simulink model "ModelGreenhouse"  (R2018a)
settings: Solver=FixedStepAuto  StartTime=0  StopTime=432000  FixedStep=5  RelTol=1e-1
undefined symbols (not defined in the file or in its folder): magnitude
libraries: simulink x6
(part 1 of 3)
settings Model: SimulationMode=accelerator  Creator=kayfr  LastModifiedBy=kayfr
settings SolverCC: MaxConsecutiveMinStep=100  AlgebraicLoopSolver=LineSearch
settings DebuggingCC: IgnoredZcDiagnostic=none

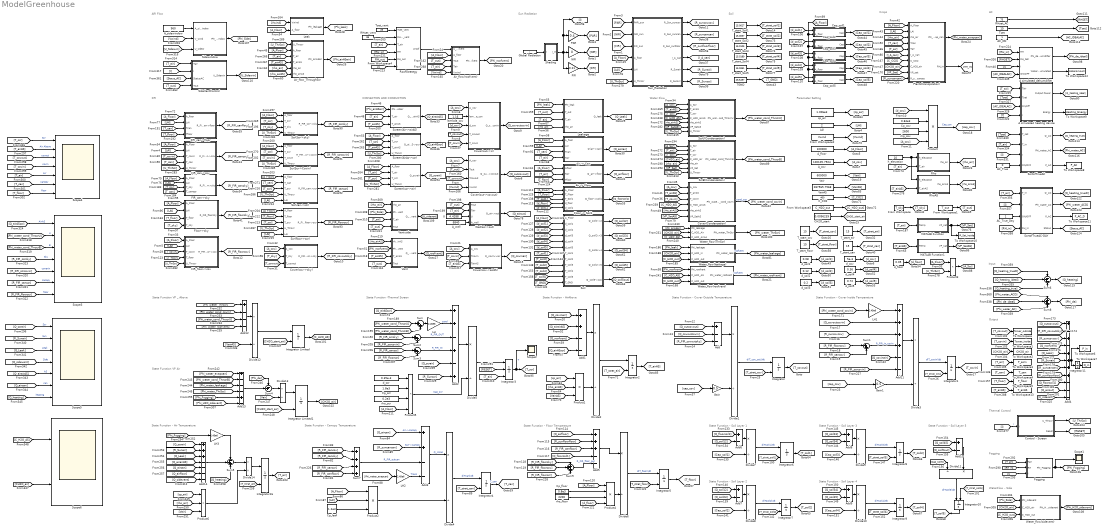
== system ModelGreenhouse ==
  note: Input
  note: AC
  note: WaterFlow - Side
  note: Fogging
  note: Thermal Control
  note: State Function - Air Temperature
  note: State Function VP Air
  note: State Function VP _ Above
  note: Crops
  note: State Function -Thermal Screen
  note: State Function - AirAbove
  note: Output
  note: State Function - Soil Layer 5
  note: State Function - Soil Layer 1
  note: Parameter Setting
  note: Soil
  note: Sun Radiation
  note: AIR Flow
  note: Water Flow
  note: CONVECTION AND CONDUCTION
  note: FIR
  note: State Function - Cover Inside Temperature
  note: State Function - Cover Outside Temperature
  note: State Function - Canopy Temperature
  note: State Function - Floor Temperature
  note: State Function - Soil Layer 2
  note: State Function - Soil Layer 3
  note: State Function - Soil Layer 4
  A simulated dehumdifier : Subsystem
  A simulated heating device : Subsystem
  AC_ON : Constant
  AC_True : Constant  Value=0
  AC_True_Day : Constant
  A_cov : Constant  Value=100105.7924
  A_floor : Constant  Value=100000
  A_sidewindow : Constant  Value=960
  A_wall : Constant  Value=6840
  Add : Sum  Inputs=+--
  Add1 : Sum  Inputs=++--
  Add{6..10} (5 alike) : Sum  Inputs=+-
  Add11 : Sum  Inputs=++++--
  Add12 : Sum  Inputs=+---
  Add13 : Sum  Inputs=+---+-
  Add14 : Sum  Inputs=+++----
  Add2 : Sum  Inputs=++-+-+
  Add3 : Sum  Inputs=++--
  Add4 : Sum  Inputs=+-+-++++---
  Add5 : Sum  Inputs=+++--
  "Air -> Can" : Subsystem
  "Air -> Floor" : Subsystem
  Air_flow(roofvent) : Subsystem
  Air_flow_ThroughScr : Subsystem
  CH2O_start : Constant  Value=0.0096239
  C_CO2 : Constant  Value=400
  Cap_soil1 : Subsystem
  Cap_soil2 : Subsystem
  Cap_soil3 : Subsystem
  Cap_soil4 : Subsystem
  Cap_soil5 : Subsystem
  Control - Screen : Subsystem
  Cover(Condensation) : Subsystem
  Cover(cov->airAS) : Subsystem
  Cover(cov->sky) : Subsystem
  Cover(out->covout) : Subsystem
  Cover(out->in) : Subsystem
  Cp_cov : Constant  Value=0.84e3
  Cp_floor : Constant  Value=0.8e3
  Cp_leaf : Constant  Value=1.2e3
  Cp_scr : Constant  Value=1.8e3
  Divide{1..10,12..14} (13 alike) : Product  Inputs=*/
  Divide11 : Product  Inputs=/*
  FIR : Gain  Gain=0.21
  FIR_can->cov : Subsystem
  FIR_can->floor : Subsystem
  FIR_can->sky : Subsystem
  FIR_floor->cov : Subsystem
  "Floor -> Soil1" : Subsystem
  Floor->sky : Subsystem
  Fogging : Subsystem
  From Workspace : FromWorkspace  VariableName=T_sky  SampleTime=0
  From Workspace1 : FromWorkspace  VariableName=T_out  SampleTime=0
  From Workspace2 : FromWorkspace  VariableName=Vwind  SampleTime=0
  From Workspace3 : FromWorkspace  VariableName=C_H2O_out  SampleTime=0
  From Workspace4 : FromWorkspace  VariableName=RH_out  SampleTime=0
  Gain : Gain  Gain=0.5
  Gain1 : Gain  Gain=0.5
  Global Radiation : FromWorkspace  VariableName=I  SampleTime=0
  Integrator{,2,4,6..10,16} (9 alike) : Integrator  InitialConditionSource=external
  Integrator Limited : Integrator  InitialConditionSource=external  LimitOutput=on  UpperSaturationLimit=100  LowerSaturationLimit=0
  Integrator Limited1 : Integrator  InitialConditionSource=external  LimitOutput=on  UpperSaturationLimit=100  LowerSaturationLimit=0
  Integrator1 : Integrator  InitialConditionSource=external  ContinuousStateAttributes='Tcov_out'
  Integrator11 : Integrator
  Integrator3 : Integrator  ExternalReset=rising  InitialConditionSource=external
  Integrator5 : Integrator  InitialConditionSource=external  ContinuousStateAttributes='T_floor'
  LAI : Constant  Value=2
  LH{,1..3} (4 alike) : Gain  Gain=2.45e6
  Leak : Subsystem
  Leakage : Subsystem
  MATLAB Function : MATLAB Function  TreatAsAtomicUnit=on
  MATLAB Function1 : MATLAB Function  TreatAsAtomicUnit=on
  NIR : Gain  Gain=0
  PAR : Gain  Gain=0.4
  Plants(transpiration) : Subsystem
  Product : Product  Inputs=4
  Product1 : Product  Inputs=3
  Product2 : Product  Inputs=3
  Product3 : Product
  Product4 : Product  Inputs=4
  Product5 : Product  Inputs=4
  Product6 : Product  Inputs=3
  RHset_AC : Constant  Value=75
  RHset_vent : Constant  Value=85
  Rho : Subsystem
  RhoAS : Subsystem
  RoofStrategy : Subsystem
  Scope1 : Scope
  Scope2 : Scope
  Scope3 : Scope  NumInputPorts=7
  Scope4 : Scope  NumInputPorts=7
  Scope5 : Scope  NumInputPorts=7
  Scope6 : Scope  NumInputPorts=2
  Scr(Scr->Covin) : Subsystem
  Scr(Scr->sky) : Subsystem
  Scr(can->scr) : Subsystem
  Scr(floor->scr) : Subsystem
  ScrB(Condensation) : Subsystem
  ScrU(Condensation) : Subsystem
  Screen(Air->airAS) : Subsystem
  Screen(AirAs->scr) : Subsystem
  Screen(scr->air) : Subsystem
  Shading : Subsystem
  SideVentControl : Subsystem
  Sidewindow : Subsystem
  Soil : Subsystem
  SortofTrueAC : Subsystem
  SortofTrueAC-DAY : Subsystem
  Sum{,1..3} (4 alike) : Sum  Inputs=|++
  Sum4 : Sum  Inputs=-+|
  Sum5 : Sum  Inputs=-++
  Sum6 : Sum  Inputs=-+-
  Sum7 : Sum  Inputs=++|++
  Sum8 : Sum  Inputs=+++
  Sum9 : Sum  Inputs=+++
  Sun_Radiation : Subsystem
  TGND : Constant  Value=26.5497
  T_start_Soil1 : Constant  Value=15.0027
  T_start_Soil2 : Constant  Value=15.0057
  T_start_Soil3 : Constant  Value=15.0105
  T_start_Soil4 : Constant  Value=15.0189
  T_start_Soil5 : Constant  Value=15.0351
  T_start_air : Constant  Value=15
  T_start_can : Constant  Value=15
  T_start_cov : Constant  Value=15
  T_start_floor : Constant  Value=15
  To Workspace : ToWorkspace  VariableName=Tcover_outside  SaveFormat=Timeseries  SampleTime=-1
  To Workspace1 : ToWorkspace  VariableName=Tcover_inside  SaveFormat=Timeseries  SampleTime=-1
  To Workspace10 : ToWorkspace  VariableName=VP_Sat_Inside  SaveFormat=Timeseries  SampleTime=-1
  To Workspace11 : ToWorkspace  VariableName=P_AC_D  SaveFormat=Timeseries  SampleTime=-1
  To Workspace12 : ToWorkspace  VariableName=WaterAmount  SaveFormat=Timeseries  SampleTime=-1
  To Workspace13 : ToWorkspace  VariableName=T_airAS  SaveFormat=Timeseries  SampleTime=-1
  To Workspace2 : ToWorkspace  VariableName=CH2O_air  SaveFormat=Timeseries  SampleTime=-1
  To Workspace3 : ToWorkspace  VariableName=T_airin  SaveFormat=Timeseries  SampleTime=-1
  To Workspace4 : ToWorkspace  VariableName=T_can  SaveFormat=Timeseries  SampleTime=-1
  To Workspace5 : ToWorkspace  VariableName=T_floor  SaveFormat=Timeseries  SampleTime=-1
  To Workspace6 : ToWorkspace  VariableName=P_in  SaveFormat=Timeseries  SampleTime=-1
  To Workspace7 : ToWorkspace  VariableName=Q_in  SaveFormat=Timeseries  SampleTime=-1
  To Workspace8 : ToWorkspace  VariableName=P_AC  SaveFormat=Timeseries  SampleTime=-1
  To Workspace9 : ToWorkspace  VariableName=Heating_Energy  SaveFormat=Timeseries  SampleTime=-1
  Tset : Constant  Value=15
  Tset_vent : Constant  Value=25
  U : Constant  Value=4.4288
  Vair : Constant  Value=600000
  VairAS : Constant  Value=287565.7568
  Vent : Subsystem
  Vent-side : Subsystem
  Wall(air->out) : Subsystem
  Water_flow(ThrScr) : Subsystem
  Water_flow(leakage) : Subsystem
  Water_flow(roofvent) : Subsystem
  Water_flow(sidevent) : Subsystem
  cp_air : Constant  Value=1.006e3
  d_cov : Constant  Value=5e-3
  d_floor : Constant  Value=0.05
  d_scr : Constant  Value=0.35e-3
  d_soil1 : Constant  Value=0.08
  d_soil2 : Constant  Value=0.12
  d_soil3 : Constant  Value=0.2
  d_soil4 : Constant  Value=0.36
  d_soil5 : Constant  Value=0.72
  h_elevation : Constant  Value=10
  lambda_cov : Constant  Value=1.16
  rho_floor : Constant  Value=2200
  rho_scr : Constant  Value=0.2e3
  rhp_cov : Constant  Value=2600
  wires:
  Divide1/1 -> Integrator/1  "d(T_cov_out)/dt"
  [T_covout] -> Cover(out->covout)/3(Tcovout)
  Cover(Condensation)/1(Phi_water_cond_covin) -> [Phi_water_cond_covin]  "cond_cov"
  NIR/1 -> [NIR]
  FIR/1 -> [FIR]
  PAR/1 -> [PAR]
  LAI/1 -> [LAI]
  [LAI] -> FIR_can->cov/2(LAI)
  [LAI] -> FIR_floor->cov/2(LAI)
  A_floor/1 -> [A_Floor]
  [A_cov] -> Cover(out->in)/1(A_cov)
  [A_cov] -> Cover(out->covout)/1(A_cov)
  [d_cov] -> Cover(out->in)/3(d_cov)
  lambda_cov/1 -> Cover(out->in)/2(lambda_cov)
  [T_covout] -> Cover(out->in)/4(T_covout)
  d_cov/1 -> [d_cov]
  Add/1 -> Divide1/1
  Gain/1 -> Divide1/2
  Cover(out->covout)/1(Q_out->covout) -> [Q_outcovout]
  Cover(out->in)/1(Q_covout->covin) -> [Q_covoutcovin]
  [Q_covoutcovin] -> Add/2
  [R_FIR_covoutsky] -> Add/3
  FIR_can->cov/1(R_FIR_can->cov) -> [R_FIR_cancov]
  [R_FIR_floorcov] -> Sum1/1
  [R_FIR_cancov] -> Sum1/2
  [A_cov] -> Cover(cov->airAS)/1(A_cov)
  Cover(cov->airAS)/1(Q_covin->air) -> [Q_covinair]
  Gain1/1 -> Divide3/2
  Divide3/1 -> Integrator1/1  "d(T_covin)/dt"
  T_start_cov/1 -> [T_strat_cov]
  Integrator1/1 -> [T_covin]
  [T_covin] -> Cover(out->in)/5(T_covin)
  [T_covin] -> Cover(cov->airAS)/2(Tcovin)
  [T_covin] -> FIR_floor->cov/3(T_covin)
  [T_covin] -> FIR_can->cov/3(T_covin)
  [T_covout] -> Cover(cov->sky)/3(T_covout)
  [A_cov] -> Cover(cov->sky)/1(A_cov)
  [A_Floor] -> FIR_floor->cov/1(A_Floor)
  [A_Floor] -> FIR_can->cov/1(A_Floor)
  [A_cov] -> Cover(Condensation)/1(A_cov)
  [T_covin] -> Cover(Condensation)/3(T_covin)
  Product/1 -> [cap_cov]  "Cap_cov"
  Cp_cov/1 -> Product/2
  [A_cov] -> Product/4
  [d_cov] -> Product/1
  rhp_cov/1 -> Product/3
  [cap_cov] -> Gain/1
  [cap_cov] -> Gain1/1
  Vair/1 -> [Vair]
  [A_Floor] -> Air_flow(roofvent)/2(A_floor)
  Air_flow(roofvent)/1(Phi_roofvent) -> [Phi_roofvent]
  [Phi_roofvent] -> Water_flow(roofvent)/1(Phi_roofvent)
  h_elevation/1 -> RhoAS/1(h_elevation), Rho/1(h_elevation)
  Rho/1(rho_air) -> [rho_air]
  [rho_airAS] -> Cover(Condensation)/5(rho_airAS)
  [A_Floor] -> Plants(transpiration)/1(A_Floor)
  [LAI] -> Plants(transpiration)/2(LAI)
  [rho_air] -> Plants(transpiration)/3(rho_air)
  [CH2O_air] -> Plants(transpiration)/8(C_H20_air)
  [C_H2O_AS] -> Water_flow(roofvent)/2(C_H2O_AS)
  [C_H2O_AS] -> Cover(Condensation)/4(C_H2O_airAS)
  [rho_airAS] -> Vent/1(rho_airAS)
  [Phi_roofvent] -> Vent/2(Phi_roofvent)
  Vent/1(Q_roofvent) -> [Q_roofvent]
  [A_Floor] -> Leak/2(A_floor)
  Leak/1(Phi_leakage) -> [Phi_leak]
  [A_Floor] -> "Air -> Can"/1(A_floor)
  [LAI] -> "Air -> Can"/2(LAI)
  "Air -> Can"/1(Q(air->can)) -> [Q_aircan]
  [A_Floor] -> "Air -> Floor"/1(Afloor)
  "Air -> Floor"/1(Q_air->floor) -> [Q_airfloor]
  T_start_air/1 -> [T_strat_air]
  [T_airAS] -> Cover(Condensation)/2(T_airAS)
  [T_air] -> Plants(transpiration)/5(Tair)
  [T_air] -> "Air -> Can"/4(Tair)
  [T_air] -> "Air -> Floor"/2(Tair)
  [T_airAS] -> Cover(cov->airAS)/3(TairAS)
  [T_airAS] -> Vent/3(T_airAS)
  [T_air] -> Rho/2(T_air)
  [A_Floor] -> FIR_can->sky/1(A_Floor)
  [LAI] -> FIR_can->sky/2(LAI)
  FIR_can->sky/1(R_FIR_can->sky) -> [R_FIR_cansky]
  [A_Floor] -> FIR_can->floor/1(A_floor)
  [LAI] -> FIR_can->floor/2(LAI)
  FIR_can->floor/1(R_FIR_can->floor) -> [R_FIR_canfloor]
  [FIR] -> Sun_Radiation/3(FIR_sun)
  [NIR] -> Sun_Radiation/2(NIR_sun)
  [PAR] -> Sun_Radiation/1(PAR_sun)
  Sun_Radiation/1(R_Sun_suncov) -> [R_suncovcov]
  [A_Floor] -> Sun_Radiation/4(A_floor)
  [LAI] -> Sun_Radiation/5(LAI)
  [I_A_can] -> Plants(transpiration)/6(I_A_can)
  Sun_Radiation/2(R_Sun_suncan) -> [R_suncancan]
  [R_FIR_cancov] -> Sum7/1
  Sum7/1 -> Add3/3  "R_FIR_outcan"
  [Q_aircan] -> Add3/1  "Air->canopy"
  [R_suncancan] -> Add3/2  "Sun->canopy"
  Product2/1 -> Divide4/2
  [A_Floor] -> Product2/1
  [LAI] -> Product2/2
  Cp_leaf/1 -> Product2/3
  Divide4/1 -> Integrator4/1  "d(Tcan)/dt"
  T_start_can/1 -> [T_strat_can]
  [T_can] -> FIR_can->cov/4(T_can)
  [T_can] -> "Air -> Can"/3(Tcan)
  [T_can] -> Plants(transpiration)/4(Tcan)
  Floor->sky/1(R_FIR_floorsky) -> [R_FIR_floorsky]
  [A_Floor] -> Floor->sky/1(A_Floor)
  [LAI] -> Floor->sky/2(LAI)
  Sun_Radiation/4(I_A_can) -> [I_A_can]
  From Workspace/1 -> [T_sky]
  [T_sky] -> Floor->sky/4(T_sky)
  [T_sky] -> Cover(cov->sky)/2(T_sky)
  TGND/1 -> [T_GND]
  [A_Floor] -> Cap_soil1/2(A_floor), Cap_soil2/2(A_floor), Cap_soil3/2(A_floor), Cap_soil4/2(A_floor), Cap_soil5/2(A_floor)
  Cap_soil1/1(Cap) -> [Cap_soil1]
  Cap_soil2/1(Cap) -> [Cap_soil2]
  Cap_soil3/1(Cap) -> [Cap_soil3]
  Cap_soil4/1(Cap) -> [Cap_soil4]
  Cap_soil5/1(Cap) -> [Cap_soil5]
  d_soil1/1 -> [d_soil1]
  d_soil2/1 -> [d_soil2]
  d_soil3/1 -> [d_soil3]
  d_soil4/1 -> [d_soil4]
  d_soil5/1 -> [d_soil5]
  d_floor/1 -> [d_floor]
  [d_soil1] -> Cap_soil1/1(d)
  [d_soil5] -> Cap_soil5/1(d)
  [d_soil4] -> Cap_soil4/1(d)
  [d_soil3] -> Cap_soil3/1(d)
  [d_soil2] -> Cap_soil2/1(d)
  [A_Floor] -> "Floor -> Soil1"/1(A_Floor)
  [d_floor] -> "Floor -> Soil1"/4(d_floor)
  [d_soil1] -> "Floor -> Soil1"/5(d_soil1)
  "Floor -> Soil1"/1(Q_floor->soil1) -> [Q_floorsoil1]
  Sun_Radiation/3(R_Sun_sunfloor) -> [R_sunfloorfloor]
  Sum9/1 -> Add5/5  "R_FIR_floor_out"
  [Q_airfloor] -> Add5/1
  [R_sunfloorfloor] -> Add5/2
  [R_FIR_canfloor] -> Add5/3
  [Q_floorsoil1] -> Add5/4
  Add5/1 -> Divide6/1
  Product4/1 -> Divide6/2
  [A_Floor] -> Product4/1
  Cp_floor/1 -> Product4/2
  rho_floor/1 -> Product4/3
  [d_floor] -> Product4/4
  Divide6/1 -> Integrator5/1  "d(T_floor)/dt"
  T_start_floor/1 -> [T_strat_floor]
  [T_floor] -> FIR_floor->cov/4(T_floor)
  [T_floor] -> "Air -> Floor"/3(Tfloor)
  [T_floor] -> "Floor -> Soil1"/2(T_Floor)
  CH2O_start/1 -> [CH2O_start_air]
  [Phi_leak] -> Leakage/1(Phi_leak)
  [T_air] -> Leakage/3(T_air)
  [rho_air] -> Leakage/4(rho_air)
  Leakage/1(Q_leak) -> [Q_Leak]
  [A_Floor] -> Soil/1(A_Floor)
  [d_soil1] -> Soil/2(d_soil1)
  [d_soil2] -> Soil/3(d_soil2)
  [d_soil3] -> Soil/4(d_soil3)
  [d_soil4] -> Soil/5(d_soil4)
  [d_soil5] -> Soil/6(d_soil5)
  Soil/1(Q_soil1->2) -> [Q_soil12]
  Soil/2(Q_soil2->3) -> [Q_soil23]
  Soil/3(Q_soil3->4) -> [Q_soil34]
  Soil/4(Q_soil4->5) -> [Q_soil45]
  Soil/5(Q_soil5->out) -> [Q_soil5out]
  [T_GND] -> Soil/12(T_GND)
  [Q_floorsoil1] -> Add6/1
  [Q_soil12] -> Add6/2
  Add6/1 -> Divide7/1
  [Cap_soil1] -> Divide7/2
  Divide7/1 -> Integrator6/1  "d(Tsoil1)/dt"
  [T_soil1] -> Soil/7(T_soil1)
  [T_soil1] -> "Floor -> Soil1"/3(T_Soil1)
  Add7/1 -> Divide8/1
  Integrator7/1 -> [T_soil2]
  [Q_soil12] -> Add7/1
  [Cap_soil2] -> Divide8/2
  Divide8/1 -> Integrator7/1  "d(Tsoil2)/dt"
  [Q_soil23] -> Add7/2
  [T_soil2] -> Soil/8(T_soil2)
  Divide9/1 -> Integrator8/1  "d(Tsoil3)/dt"
  [Cap_soil3] -> Divide9/2
  [Q_soil34] -> Add8/2
  [Q_soil23] -> Add8/1
  Add8/1 -> Divide9/1
  [T_soil3] -> Soil/9(T_soil3)
  Divide10/1 -> Integrator9/1  "d(Tsoil4)/dt"
  [Cap_soil4] -> Divide10/2
  [Q_soil45] -> Add9/2
  [Q_soil34] -> Add9/1
  Add9/1 -> Divide10/1
  [T_soil4] -> Soil/10(T_soil4)
  [Q_soil45] -> Add10/1
  [Q_soil5out] -> Add10/2
  Add10/1 -> Divide11/2
  [Cap_soil5] -> Divide11/1
  Divide11/1 -> Integrator10/1  "d(Tsoil5)/dt"
  [T_soil5] -> Soil/11(T_soil5)
  From Workspace1/1 -> [T_out]
  [T_out] -> Leakage/2(T_out)
  [T_out] -> Cover(out->covout)/2(Tout)
  [T_out] -> Vent/4(Tout)
  [T_out] -> Air_flow(roofvent)/3(Tout)
  [T_floor] -> Floor->sky/3(T_floor)
  From Workspace2/1 -> [Vwind]
  [Vwind] -> Leak/1(Vwind)
  [Vwind] -> Air_flow(roofvent)/5("Vwind ")
  RoofStrategy/1(Uroof) -> Air_flow(roofvent)/1(U_roofvent)
  [Vwind] -> Cover(out->covout)/4(Vwind)
  C_CO2/1 -> [C_CO2]
  [C_CO2] -> Plants(transpiration)/7(C_CO2)
  From Workspace3/1 -> [C_H2O_out]
  [C_H2O_out] -> Water_flow(roofvent)/3(C_H2O_out)
  T_start_Soil2/1 -> [T_strat_soil2]
  T_start_Soil3/1 -> [T_strat_soil3]
  T_start_Soil4/1 -> [T_strat_soil4]
  [VP_Sat] -> Plants(transpiration)/9(VP_sat)
  Cover(cov->sky)/1(R_FIR_covout->sky) -> [R_FIR_covoutsky]
  FIR_floor->cov/1(R_FIR_floor->cov) -> [R_FIR_floorcov]
  [Q_outcovout] -> Add/1
  [Phi_water_cond_covin] -> LH1/1
  Add11/1 -> Divide3/1
  LH1/1 -> Add11/1
  [Q_covoutcovin] -> Add11/2
  [R_suncovcov] -> Add11/3
  Sum1/1 -> Add11/4  "R_FIR_in_covin"
  [Q_covinair] -> Add11/5
  [T_strat_cov] -> Integrator1/2
  Integrator/1 -> [T_covout]
  [T_strat_cov] -> Integrator/2
  Integrator4/1 -> [T_can]  "T_can"
  [T_strat_can] -> Integrator4/2
  [T_strat_floor] -> Integrator5/2
  Integrator5/1 -> [T_floor]
  [T_strat_soil1] -> Integrator6/2
  Integrator6/1 -> [T_soil1]
  [T_strat_soil2] -> Integrator7/2
  Integrator8/1 -> [T_soil3]
  [T_strat_soil3] -> Integrator8/2
  [T_strat_soil4] -> Integrator9/2
  Integrator9/1 -> [T_soil4]
  [T_strat_soil5] -> Integrator10/2
  Integrator10/1 -> [T_soil5]
  Water_flow(roofvent)/1(Phi_water_roofvent) -> [Phi_water_roofvent]  "roofvent"
  [T_can] -> FIR_can->floor/3(Tcan)
  [T_floor] -> FIR_can->floor/4(Tfloor)
  T_start_Soil1/1 -> [T_strat_soil1]
  T_start_Soil5/1 -> [T_strat_soil5]
  [T_covout] -> To Workspace/1
  [T_covin] -> To Workspace1/1
  [CH2O_air] -> To Workspace2/1
  [T_air] -> To Workspace3/1
  [T_can] -> To Workspace4/1
  [T_floor] -> To Workspace5/1
  Add4/1 -> To Workspace6/1, Integrator11/1
  Integrator11/1 -> To Workspace7/1
  Sun_Radiation/5(R_Sunair) -> [R_Sunair]
  [Q_outcovout] -> Add4/1
  [R_FIR_covoutsky] -> Add4/2
  [R_suncovcov] -> Add4/3
  [Q_roofvent] -> Add4/4
  [Q_Leak] -> Add4/5
  [R_Sunair] -> Add4/6
  [R_suncancan] -> Add4/7
  [R_sunfloorfloor] -> Add4/8
  [Q_floorsoil1] -> Add4/9
  [T_sky] -> FIR_can->sky/3(T_sky)
  [T_can] -> FIR_can->sky/4(T_canopy)
  [T_out] -> Wall(air->out)/1(Tout)
  [T_air] -> Wall(air->out)/2(Tair)
  U/1 -> Wall(air->out)/3(U)
  A_wall/1 -> Wall(air->out)/4(A_wall)
  Wall(air->out)/1(Q_air->out) -> [Q_airout]
  [Q_airout] -> Add4/10
  LH2/1 -> Add3/4  "Trans"
  [T_air] -> MATLAB Function/1(Temp)
  MATLAB Function/1(VP_sat) -> [VP_Sat], To Workspace10/1
  Add3/1 -> Divide4/1  "Q_incan"
  A_cov/1 -> [A_cov]
  Water_flow(leakage)/1(Phi_water_leak) -> [Phi_water_leakage]  "roofvent"
  [Phi_leak] -> Water_flow(leakage)/1(Phi_leakage)
  [CH2O_air] -> Water_flow(leakage)/2(C_H2O_in)
  [C_H2O_out] -> Water_flow(leakage)/3(C_H2O_out)
  [A_Floor] -> Air_flow_ThroughScr/2(A_floor)
  Air_flow_ThroughScr/1(Phi_airASair) -> [Phi_airASair]
  [Phi_airASair] -> Screen(Air->airAS)/1(Phi_airASair)
  Screen(Air->airAS)/1(Q_air->airAS) -> [Q_airairAS]
  [A_Floor] -> Screen(AirAs->scr)/1(A_floor)
  Screen(AirAs->scr)/1(Q_airAS->scr) -> [Q_airASscr]
  [Q_covinair] -> Add1/1
  [Q_roofvent] -> Add1/3
  [Q_airairAS] -> Add1/2
  [Q_airASscr] -> Add1/4
  Add1/1 -> Divide2/1
  RhoAS/1(rho_airAS) -> [rho_airAS]
  [rho_airAS] -> Air_flow_ThroughScr/6(rho_airAS)
  [rho_air] -> Air_flow_ThroughScr/5(rho_air)
  VairAS/1 -> [VairAS]
  cp_air/1 -> [cp_air]
  [cp_air] -> Product1/1
  [rho_airAS] -> Product1/2
  [VairAS] -> Product1/3
  Product1/1 -> Divide2/2
  Divide2/1 -> Integrator2/1
  [T_strat_air] -> Integrator2/2
  Integrator2/1 -> [T_airAS]
  MATLAB Function1/1(VP_sat) -> [VP_SatAS]
  [T_airAS] -> MATLAB Function1/1(Temp)
  [VP_SatAS] -> Cover(Condensation)/6(VP_SatAS)
  ScrU(Condensation)/1(Phi_water_cond_ThrscrU) -> [Phi_water_cond_ThrscrU]
  [A_Floor] -> Product3/1
  Product3/1 -> [A_Scr]
  [A_Scr] -> ScrU(Condensation)/1(A_Scr)
  [T_airAS] -> ScrU(Condensation)/2(T_airAS)
  [rho_airAS] -> ScrU(Condensation)/5(rho_airAS)
  [VP_SatAS] -> ScrU(Condensation)/6(VP_SatAS)
  [rho_air] -> ScrB(Condensation)/5(rho_air)
  [VP_Sat] -> ScrB(Condensation)/6(VP_Sat)
  [A_Scr] -> ScrB(Condensation)/1(A_Scr)
  ScrB(Condensation)/1(Phi_water_cond_ThrscrB) -> [Phi_water_cond_ThrscrB]
  [Phi_water_cond_ThrscrU] -> Sum/1
  [Phi_water_cond_ThrscrB] -> Sum/2
  Sum/1 -> LH/1
  Scr(Scr->sky)/1(R_FIR_scr->sky) -> [R_FIR_scrsky]
  [T_sky] -> Scr(Scr->sky)/3(T_sky)
  [A_Floor] -> Scr(Scr->sky)/1(A_floor)
  Scr(Scr->Covin)/1(R_FIR_scr->covin) -> [R_FIR_scrcovin]
  [A_Floor] -> Scr(Scr->Covin)/1(A_floor)
  [T_covin] -> Scr(Scr->Covin)/3(T_covin)
  [A_Floor] -> Scr(can->scr)/1(A_floor)
  Scr(can->scr)/1(R_FIR_can->scr) -> [R_FIR_canscr]
  Scr(floor->scr)/1(R_FIR_floor->scr) -> [R_FIR_floorscr]
  [A_Floor] -> Scr(floor->scr)/1(A_floor)
  [R_FIR_scrsky] -> Sum2/1
  [R_FIR_scrcovin] -> Sum2/2
  [R_FIR_canscr] -> Sum3/1
  [R_FIR_floorscr] -> Sum3/2
  [A_Floor] -> Screen(scr->air)/1(A_floor)
  Screen(scr->air)/1(Q_scrair) -> [Q_scrair]
  Sum2/1 -> Add2/3  "R_FIR_OUT"
  Sum3/1 -> Add2/4  "R_FIR_IN"
  [Q_airASscr] -> Add2/1
  [Q_scrair] -> Add2/5
  Add2/1 -> Divide5/1
  rho_scr/1 -> Product5/3
  [A_Floor] -> Product5/4
  Product5/1 -> Divide5/2  "Cap_scr"
  d_scr/1 -> Product5/1
  Cp_scr/1 -> Product5/2
  Divide5/1 -> Integrator3/1
  [T_air] -> Integrator3/3
  Integrator3/1 -> Scope2/1, [T_scr]  "T"
  [T_floor] -> Scr(floor->scr)/2(T_floor)
  [T_scr] -> Scr(floor->scr)/3(T_scr)
  [LAI] -> Scr(can->scr)/5(LAI)
  [LAI] -> Scr(floor->scr)/5(LAI)
  [T_scr] -> Scr(can->scr)/3(T_scr)
  Plants(transpiration)/1(Phi_water_evap_can) -> [Phi_water_evapcan]
  [R_suncancan] -> Plants(transpiration)/10(R_suncanopy)
  Tset_vent/1 -> RoofStrategy/1(Tset_vent)
  [I] -> RoofStrategy/6(I)
  RHset_vent/1 -> RoofStrategy/2(RHset_vent)
  From Workspace4/1 -> RoofStrategy/5(RH_out)
  Plants(transpiration)/2(RH_in) -> [RH_in]
  [RH_in] -> RoofStrategy/4(RH)
  [RHSET] -> A simulated dehumdifier/2(RH_Set)
  [I] -> A simulated heating device/4(I)
  [T_air] -> A simulated heating device/1(Tair)
  [RH_in] -> A simulated dehumdifier/1(RH)
  [Tset] -> A simulated heating device/2(Tset)
  [I] -> A simulated dehumdifier/3(I)
  [R_FIR_cansky] -> Sum7/2
  [R_FIR_scrcovin] -> Add11/6
  [R_FIR_floorsky] -> Sum9/1
  [R_FIR_floorcov] -> Sum9/2
  [R_FIR_floorscr] -> Sum9/3
  Sun_Radiation/6("R_Sunscr ") -> [R_Sunscr]
  [R_Sunscr] -> Add2/6
  [Phi_airASair] -> Water_flow(ThrScr)/1(Phi_leakage)
  [CH2O_air] -> Water_flow(ThrScr)/2(C_H2O_Air)
  Water_flow(ThrScr)/1(Phi_water_ThrScr) -> [Phi_water_ThrScr]
  [Phi_water_ThrScr] -> Add12/1
  [Phi_water_cond_covin] -> Add12/2
  [Phi_water_cond_ThrscrU] -> Add12/3
  [Phi_water_roofvent] -> Add12/4
  Add12/1 -> Divide12/1
  [VairAS] -> Divide12/2
  Divide12/1 -> Integrator Limited/1
  [CH2O_start_air] -> Integrator Limited/2
  [C_H2O_AS] -> ScrU(Condensation)/4(C_H2O_airAS)
  [C_H2O_AS] -> Water_flow(ThrScr)/3(C_H2O_AirAs)
  [Phi_water_ThrScr] -> Add13/4
  [Phi_water_leakage] -> Add13/3
  [Phi_water_cond_ThrscrB] -> Add13/2
  [Phi_water_evapcan] -> Add13/1
  Add13/1 -> Sum4/2
  [Phi_de] -> Sum4/1
  Sum4/1 -> Divide13/1
  [Vair] -> Divide13/2
  Divide13/1 -> Integrator Limited1/1
  [CH2O_start_air] -> Integrator Limited1/2
  [Vair] -> Product6/3
  [rho_air] -> Product6/2
  [cp_air] -> Product6/1
  [Q_airfloor] -> Add14/6
  [Q_aircan] -> Add14/5
  [Q_airairAS] -> Add14/4
  [Q_Leak] -> Add14/3
  [R_Sunair] -> Add14/2
  [Q_scrair] -> Add14/1
  Add14/1 -> Sum5/2
  Sum5/1 -> Divide14/1
  Product6/1 -> Divide14/2
  Divide14/1 -> Integrator16/1
  [T_strat_air] -> Integrator16/2
  Integrator16/1 -> [T_air]
  [T_air] -> Screen(Air->airAS)/2(T_air)
  [T_airAS] -> Screen(Air->airAS)/3(T_airAS)
  [T_scr] -> Screen(scr->air)/3(T_scr)
  [T_scr] -> Screen(AirAs->scr)/2(T_scr)
  [T_airAS] -> Screen(AirAs->scr)/3(T_airAS)
  [T_air] -> Screen(scr->air)/2(T_air)
  [T_air] -> RoofStrategy/3(T_air)
  [T_air] -> Air_flow_ThroughScr/3(T_air)
  [T_airAS] -> Air_flow_ThroughScr/4(T_airAS)
  [T_air] -> Air_flow(roofvent)/4(Tair)
  [T_scr] -> Scr(Scr->sky)/2(T_scr)
  [T_scr] -> Scr(Scr->Covin)/2(T_scr)
  [T_can] -> Scr(can->scr)/2(T_can)
  [T_air] -> ScrB(Condensation)/2(T_air)
  [T_scr] -> ScrB(Condensation)/3(T_scr)
  [CH2O_air] -> ScrB(Condensation)/4(C_H2O_air)
  [T_scr] -> ScrU(Condensation)/3(T_scr)
  [T_airAS] -> RhoAS/2(T_airAS)
  [U_ThrScr] -> Product3/2
  [U_ThrScr] -> Sun_Radiation/6(U_Thrscr)
  [U_ThrScr] -> Screen(AirAs->scr)/4(U_Thrscr)
  [U_ThrScr] -> Screen(scr->air)/4(U_Thrscr)
  [U_ThrScr] -> FIR_floor->cov/5(U_Thrscr)
  [U_ThrScr] -> FIR_can->cov/5(U_Thrscr)
  [U_ThrScr] -> Scr(Scr->sky)/4(U_Thrscr)
  [U_ThrScr] -> Scr(Scr->Covin)/4(U_Thrscr)
  [U_ThrScr] -> Scr(can->scr)/4(U_Thrscr)
  [U_ThrScr] -> Scr(floor->scr)/4(U_Thrscr)
  [T_airAS] -> To Workspace13/1
  [U_ThrScr] -> Air_flow_ThroughScr/1(U_Thrscr)
  [I] -> Control - Screen/1(I)  "I"
  Control - Screen/1(U_Thrscr) -> [U_ThrScr]
  Control - Screen/2(Reset) -> [RESET]
  [RESET] -> Integrator3/2
  LH/1 -> Add2/2  "cond"
  [U_ThrScr] -> ScrB(Condensation)/7(U_Thrscr)
  [U_ThrScr] -> ScrU(Condensation)/7(U_Thrscr)
  [T_airAS] -> Scope4/2  "Air Above"
  [T_covout] -> Scope4/3  "covout"
  [T_covin] -> Scope4/4  "covin"
  [T_air] -> Scope4/5  "Air"
  [T_can] -> Scope4/6  "canopy"
  [T_floor] -> Scope4/7  "floor"
  A simulated heating device/1(Output Power) -> [Q_heating_ideal]
  [RH_in] -> Fogging/2(RH)
  [T_air] -> Fogging/1(Tair)
  [I] -> Fogging/3(I)
  [Q_heating] -> Sum5/3
  [Phi_Fogging] -> LH3/1
  LH3/1 -> Sum5/1
  [Phi_Fogging] -> Add13/5
  Shading/1(I_in) -> PAR/1, [I], FIR/1, NIR/1
  Global Radiation/1 -> Shading/1(I)
  Fogging/1(Phi_Fogging) -> Scope1/1, [Phi_Fogging]
  A_sidewindow/1 -> Sidewindow/1(A_sidewindow)
  [Vwind] -> Sidewindow/2(V_wind)
  Sidewindow/1(Phi_Sidewindow) -> [Phi_Side]
  [Phi_Side] -> Water_flow(sidevent)/1(Phi_sidevent)
  [CH2O_air] -> Water_flow(sidevent)/2(C_H2O_air)
  [C_H2O_out] -> Water_flow(sidevent)/3(C_H2O_out)
  Water_flow(sidevent)/1(Phi_H2O_sidevent) -> [Phi_H2O_sidevent]
  [Phi_H2O_sidevent] -> Add13/6
  [Phi_Side] -> Vent-side/2(Phi_sidevent)
  [rho_air] -> Vent-side/1(rho_air)
  [T_air] -> Vent-side/3(T_air)
  [T_out] -> Vent-side/4(Tout)
  Vent-side/1(Q_sidevent) -> [Q_sidevent]
  [Q_sidevent] -> Add14/7
  [T_air] -> SideVentControl/1(Tair)
  SideVentControl/1(U_Sidewin) -> [U_Sidewin]
  [U_Sidewin] -> Sidewindow/3(U_sidew)
  [I] -> SideVentControl/2(I)
  [R_FIR_canscr] -> Sum7/3
  [R_FIR_canfloor] -> Sum7/4
  [Phi_water_evapcan] -> LH2/1
  [Q_airASscr] -> Scope3/1  "AirAS"
  [Phi_water_cond_ThrscrU] -> Scope3/2  "U"
  [Phi_water_cond_ThrscrB] -> Scope3/3  "B"
  [R_FIR_scrsky] -> Scope3/4  "Sky"
  [R_FIR_scrcovin] -> Scope3/5  "coverin"
  [R_FIR_canscr] -> Scope3/6  "canopy"
  [R_FIR_floorscr] -> Scope3/7  "floor"
  [Q_sidevent] -> Add4/11
  RHset_AC/1 -> [RHSET]
  Tset/1 -> [Tset]
  AC_ON/1 -> [AC_IDEALAC]
  [AC_IDEALAC] -> A simulated dehumdifier/4(ON/OFF)
  A simulated heating device/2(Energy) -> To Workspace9/1
  [Tset] -> SortofTrueAC/1(T_set)
  AC_True/1 -> SortofTrueAC/4(ON/OFF)
  [I] -> SortofTrueAC/3(I)
  [T_air] -> SortofTrueAC/2(T_in)
  SortofTrueAC/1(Q_AC) -> [Q_heating_true]
  Sum6/1 -> [Q_heating]
  SortofTrueAC/2(Phi_water_AC) -> [Phi_water_AC]
  Sum8/1 -> [Phi_de]
  [AC_IDEALAC] -> A simulated heating device/3(On/Off)
  SortofTrueAC/3(P_AC) -> To Workspace8/1
  [Q_scrair] -> Scope5/1  "Scr"
  [R_Sunair] -> Scope5/2  "Sun"
  [Q_Leak] -> Scope5/3  "Leak"
  [Q_sidevent] -> Scope5/4  "Side"
  [Q_airairAS] -> Scope5/5  "AS"
  [Q_aircan] -> Scope5/6  "can"
  [Q_heating] -> Scope5/7  "heating"
  [T_scr] -> Scope4/1  "Scr"
  [CH2O_air] -> Scope6/2
  [C_H2O_AS] -> Scope6/1
  A simulated dehumdifier/1(Phi_dehumidifier) -> [Phi_de_ideal]
  A simulated dehumdifier/2(WaterAccumulated) -> To Workspace12/1
  Integrator Limited/1 -> [C_H2O_AS]
  Integrator Limited1/1 -> [CH2O_air]
  SortofTrueAC-DAY/3(P_AC) -> To Workspace11/1
  [I] -> SortofTrueAC-DAY/2(I)
  SortofTrueAC-DAY/2(Phi_water_AC) -> [Phi_water_ACD]
  SortofTrueAC-DAY/1(Q_AC) -> [Q_heating_trueD]
  AC_True_Day/1 -> SortofTrueAC-DAY/3(ON/OFF)
  [T_air] -> SortofTrueAC-DAY/1(T_in)
  [Q_heating_trueD] -> Sum6/1
  [Q_heating_ideal] -> Sum6/2
  [Q_heating_true] -> Sum6/3
  [Phi_water_AC] -> Sum8/3
  [Phi_de_ideal] -> Sum8/2
  [Phi_water_ACD] -> Sum8/1
  SortofTrueAC-DAY/4(Status) -> [Staus_AC]
  [Staus_AC] -> SideVentControl/3(StatusAC)
  [T_out] -> SideVentControl/4(Tout)
  [RH_in] -> SortofTrueAC-DAY/4(RH_in)

== system ModelGreenhouse/A simulated dehumdifier ==
  RH : Inport
  RH_Set : Inport  Port=2
  I : Inport  Port=3
  ON/OFF : Inport  Port=4
  Constant : Constant  Value=0
  Constant1 : Constant  Value=0
  Integrator12 : Integrator
  Manual Switch : ManualSwitch
  PID Controller : simulink/Continuous/PID Controller  Controller=PI  TimeDomain=Continuous-time  SampleTime=-1  IntegratorMethod=Forward Euler  FilterMethod=Forward Euler  Form=Parallel  UseFilter=on  ControllerParametersSource=internal  P=20  I=1e-8  D=0  N=100  InitialConditionSource=internal  InitialConditionForIntegrator=0  InitialConditionForFilter=0  ExternalReset=none  LimitOutput=off  UpperSaturationLimit=inf  LowerSaturationLimit=-inf  LinearizeAsGain=on  AntiWindupMode=none  Kb=1  TrackingMode=off  Kt=1  PParamMin=[]  PParamMax=[]  IParamMin=[]  IParamMax=[]  DParamMin=[]  DParamMax=[]  NParamMin=[]  NParamMax=[]  KbParamMin=[]  KbParamMax=[]  KtParamMin=[]  KtParamMax=[]  POutMin=[]  POutMax=[]  IOutMin=[]  IOutMax=[]  DOutMin=[]  DOutMax=[]  NOutMin=[]  NOutMax=[]  KbOutMin=[]  KbOutMax=[]  KtOutMin=[]  KtOutMax=[]  IntegratorOutMin=[]  IntegratorOutMax=[]  FilterOutMin=[]  FilterOutMax=[]  SumOutMin=[]  SumOutMax=[]  SumI1OutMin=[]  SumI1OutMax=[]  SumI2OutMin=[]  SumI2OutMax=[]  SumI3OutMin=[]  SumI3OutMax=[]  SumDOutMin=[]  SumDOutMax=[]  SaturationOutMin=[]  SaturationOutMax=[]  IntegratorContinuousStateAttributes=''  IntegratorStateMustResolveToSignalObject=off  IntegratorRTWStateStorageClass=Auto  FilterContinuousStateAttributes=''  FilterStateMustResolveToSignalObject=off  FilterRTWStateStorageClass=Auto  DifferentiatorICPrevScaledInput=0  DifferentiatorOutMin=[]  DifferentiatorOutMax=[]  FilterDiffOutCoefMin=[]  FilterDiffOutCoefMax=[]  SumDenOutMin=[]  SumDenOutMax=[]  SumNumOutMin=[]  SumNumOutMax=[]  ReciprocalOutMin=[]  ReciprocalOutMax=[]  DivideOutMin=[]  DivideOutMax=[]  TunerSelectOption=Transfer Function Based (PID Tuner App)
  Saturation : Saturate  UpperLimit=100  LowerLimit=0
  Scope : Scope  NumInputPorts=2
  Sum : Sum  Inputs=|+-
  Switch : Switch  Criteria=u2 > Threshold
  day/night : Switch  Criteria=u2 > Threshold  Threshold=20
  Phi_dehumidifier : Outport
  WaterAccumulated : Outport  Port=2
  wires:
  RH_Set/1 -> Sum/2
  RH/1 -> Scope/1, Sum/1
  Sum/1 -> Saturation/1
  Saturation/1 -> PID Controller/1
  I/1 -> day/night/2
  PID Controller/1 -> day/night/3
  Constant/1 -> day/night/1
  ON/OFF/1 -> Switch/2
  day/night/1 -> Switch/1
  Switch/1 -> Manual Switch/1, Scope/2
  Constant1/1 -> Manual Switch/2, Switch/3
  Integrator12/1 -> WaterAccumulated/1
  Manual Switch/1 -> Integrator12/1, Phi_dehumidifier/1

== system ModelGreenhouse/A simulated heating device ==
  note: 1GW Max
  Tair : Inport
  Tset : Inport  Port=2
  On/Off : Inport  Port=3
  I : Inport  Port=4
  Constant : Constant  Value=0
  Constant1 : Constant  Value=0
  Constant2 : Constant  Value=0
  Constant3 : Constant
  Integrator : Integrator
  PID Controller : simulink/Continuous/PID Controller  Controller=PI  TimeDomain=Continuous-time  SampleTime=-1  IntegratorMethod=Forward Euler  FilterMethod=Forward Euler  Form=Parallel  UseFilter=on  ControllerParametersSource=internal  P=200  I=100  D=0  N=100  InitialConditionSource=internal  InitialConditionForIntegrator=0  InitialConditionForFilter=0  ExternalReset=rising  IgnoreLimit=on  LimitOutput=off  UpperSaturationLimit=inf  LowerSaturationLimit=-inf  LinearizeAsGain=on  AntiWindupMode=none  Kb=1  TrackingMode=off  Kt=1  PParamMin=[]  PParamMax=[]  IParamMin=[]  IParamMax=[]  DParamMin=[]  DParamMax=[]  NParamMin=[]  NParamMax=[]  KbParamMin=[]  KbParamMax=[]  KtParamMin=[]  KtParamMax=[]  POutMin=[]  POutMax=[]  IOutMin=[]  IOutMax=[]  DOutMin=[]  DOutMax=[]  NOutMin=[]  NOutMax=[]  KbOutMin=[]  KbOutMax=[]  KtOutMin=[]  KtOutMax=[]  IntegratorOutMin=[]  IntegratorOutMax=[]  FilterOutMin=[]  FilterOutMax=[]  SumOutMin=[]  SumOutMax=[]  SumI1OutMin=[]  SumI1OutMax=[]  SumI2OutMin=[]  SumI2OutMax=[]  SumI3OutMin=[]  SumI3OutMax=[]  SumDOutMin=[]  SumDOutMax=[]  SaturationOutMin=[]  SaturationOutMax=[]  IntegratorContinuousStateAttributes=''  IntegratorStateMustResolveToSignalObject=off  IntegratorRTWStateStorageClass=Auto  FilterContinuousStateAttributes=''  FilterStateMustResolveToSignalObject=off  FilterRTWStateStorageClass=Auto  DifferentiatorICPrevScaledInput=0  DifferentiatorOutMin=[]  DifferentiatorOutMax=[]  FilterDiffOutCoefMin=[]  FilterDiffOutCoefMax=[]  SumDenOutMin=[]  SumDenOutMax=[]  SumNumOutMin=[]  SumNumOutMax=[]  ReciprocalOutMin=[]  ReciprocalOutMax=[]  DivideOutMin=[]  DivideOutMax=[]  TunerSelectOption=Transfer Function Based (PID Tuner App)
  Scope1 : Scope
  Sum : Sum  Inputs=|-+
  Switch : Switch  Criteria=u2 > Threshold
  day/night : Switch  Criteria=u2 > Threshold  Threshold=20
  day/night1 : Switch  Criteria=u2 > Threshold  Threshold=22
  Output Power : Outport
  Energy : Outport  Port=2
  wires:
  On/Off/1 -> Switch/2
  I/1 -> day/night1/2, day/night/2
  Integrator/1 -> Energy/1
  day/night/1 -> Integrator/1, Scope1/1, Output Power/1
  Constant/1 -> Switch/3
  PID Controller/1 -> Switch/1
  Constant1/1 -> day/night/1
  Switch/1 -> day/night/3
  Tair/1 -> Sum/1
  Tset/1 -> Sum/2
  Sum/1 -> PID Controller/1
  Constant2/1 -> day/night1/1
  Constant3/1 -> day/night1/3
  day/night1/1 -> PID Controller/2

== system ModelGreenhouse/Air -> Can ==
  A_floor : Inport
  LAI : Inport  Port=2
  Tcan : Inport  Port=3
  Tair : Inport  Port=4
  Gain : Gain  Gain=2
  Product : Product
  Product1 : Product  Inputs=3
  Sum : Sum  Inputs=|+-
  alpha_airleaf : Constant  Value=5
  Q(air->can) : Outport
  wires:
  LAI/1 -> Gain/1
  A_floor/1 -> Product/1
  Gain/1 -> Product/2
  alpha_airleaf/1 -> Product1/1
  Product/1 -> Product1/2
  Sum/1 -> Product1/3
  Tair/1 -> Sum/1
  Tcan/1 -> Sum/2
  Product1/1 -> Q(air->can)/1

== system ModelGreenhouse/Air -> Floor ==
  Afloor : Inport
  Tair : Inport  Port=2
  Tfloor : Inport  Port=3
  Fcn : Fcn  Expr=abs(u)^0.33
  Gain : Gain  Gain=1.7
  Gain1 : Gain  Gain=1.3
  MATLAB Function2 : MATLAB Function  TreatAsAtomicUnit=on
  Product : Product  Inputs=3
  Sum : Sum  Inputs=|+-
  Q_air->floor : Outport
  wires:
  Tfloor/1 -> MATLAB Function2/4(key), Sum/2
  Tair/1 -> Sum/1, MATLAB Function2/3(thres)
  Sum/1 -> Product/2, Fcn/1
  Gain/1 -> MATLAB Function2/1(u_upper)
  Gain1/1 -> MATLAB Function2/2(u_lower)
  Fcn/1 -> Gain/1, Gain1/1
  MATLAB Function2/1(Out) -> Product/3  "K"
  Afloor/1 -> Product/1
  Product/1 -> Q_air->floor/1

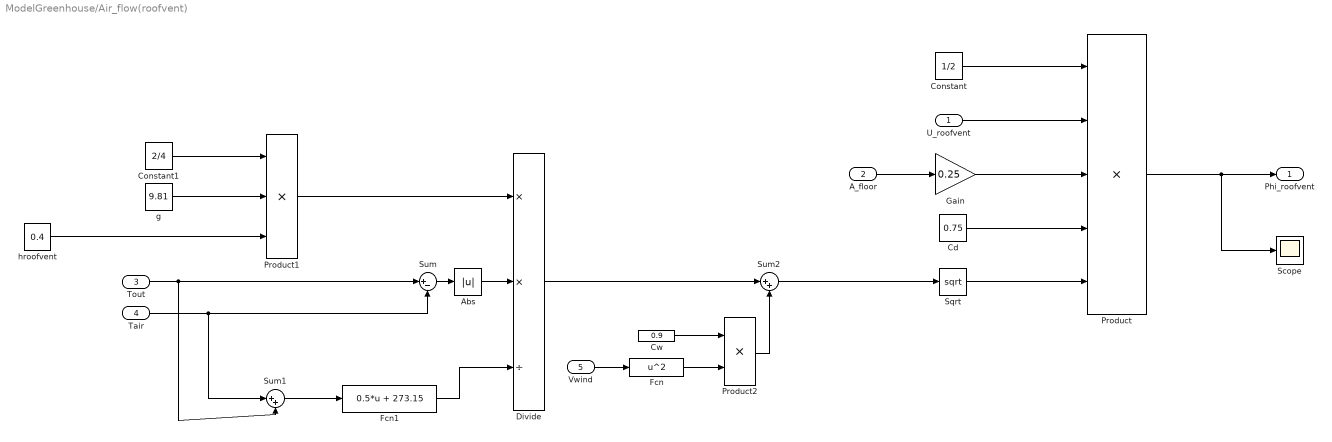
== system ModelGreenhouse/Air_flow(roofvent) ==
  U_roofvent : Inport
  A_floor : Inport  Port=2
  Tout : Inport  Port=3
  Tair : Inport  Port=4
  "Vwind " : Inport  Port=5
  Abs : Abs
  Cd : Constant  Value=0.75
  Constant : Constant  Value=1/2
  Constant1 : Constant  Value=2/4
  Cw : Constant  Value=0.9
  Divide : Product  Inputs=**/
  Fcn : Fcn  Expr=u^2
  Fcn1 : Fcn  Expr=0.5*u + 273.15
  Gain : Gain  Gain=0.25
  Product : Product  Inputs=5
  Product1 : Product  Inputs=3
  Product2 : Product
  Scope : Scope
  Sqrt : Sqrt  SaturateOnIntegerOverflow=on
  Sum : Sum  Inputs=|+-
  Sum1 : Sum  Inputs=|++
  Sum2 : Sum  Inputs=|++
  "g " : Constant  Value=9.81
  hroofvent : Constant  Value=0.4
  Phi_roofvent : Outport
  wires:
  A_floor/1 -> Gain/1
  Constant/1 -> Product/1
  U_roofvent/1 -> Product/2
  Gain/1 -> Product/3
  Cd/1 -> Product/4
  Tout/1 -> Sum/1, Sum1/2
  Tair/1 -> Sum/2, Sum1/1
  Sum/1 -> Abs/1
  Abs/1 -> Divide/2
  "g "/1 -> Product1/2
  Constant1/1 -> Product1/1
  hroofvent/1 -> Product1/3
  Product1/1 -> Divide/1
  Divide/1 -> Sum2/1
  "Vwind "/1 -> Fcn/1
  Cw/1 -> Product2/1
  Fcn/1 -> Product2/2
  Product2/1 -> Sum2/2
  Sum2/1 -> Sqrt/1
  Sqrt/1 -> Product/5
  Product/1 -> Scope/1, Phi_roofvent/1
  Fcn1/1 -> Divide/3
  Sum1/1 -> Fcn1/1

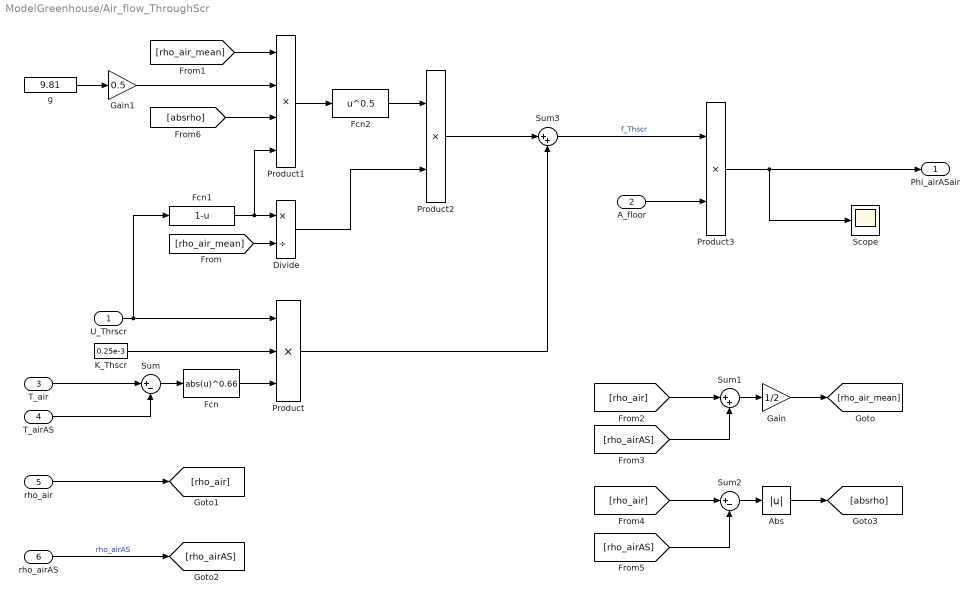
== system ModelGreenhouse/Air_flow_ThroughScr ==
  U_Thrscr : Inport
  A_floor : Inport  Port=2
  T_air : Inport  Port=3
  T_airAS : Inport  Port=4
  rho_air : Inport  Port=5
  rho_airAS : Inport  Port=6
  Abs : Abs
  Divide : Product  Inputs=*/
  Fcn : Fcn  Expr=abs(u)^0.66
  Fcn1 : Fcn  Expr=1-u
  Fcn2 : Fcn  Expr=u^0.5
  Gain : Gain  Gain=1/2
  Gain1 : Gain  Gain=0.5
  K_Thscr : Constant  Value=0.25e-3
  Product : Product  Inputs=3
  Product1 : Product  Inputs=4
  Product2 : Product
  Product3 : Product
  Scope : Scope
  Sum : Sum  Inputs=|+-
  Sum1 : Sum  Inputs=|++
  Sum2 : Sum  Inputs=|+-
  Sum3 : Sum  Inputs=|++
  g : Constant  Value=9.81
  Phi_airASair : Outport
  wires:
  T_air/1 -> Sum/1
  T_airAS/1 -> Sum/2
  Sum/1 -> Fcn/1
  U_Thrscr/1 -> Fcn1/1, Product/1
  K_Thscr/1 -> Product/2
  Fcn/1 -> Product/3
  Sum1/1 -> Gain/1
  Gain/1 -> [rho_air_mean]
  Fcn1/1 -> Product1/4, Divide/1
  [rho_air_mean] -> Divide/2
  [rho_air_mean] -> Product1/1
  rho_airAS/1 -> [rho_airAS]  "rho_airAS"
  [rho_air] -> Sum1/1
  [rho_airAS] -> Sum1/2
  [rho_air] -> Sum2/1
  [rho_airAS] -> Sum2/2
  Sum2/1 -> Abs/1
  Abs/1 -> [absrho]
  [absrho] -> Product1/3
  Gain1/1 -> Product1/2
  g/1 -> Gain1/1
  Product1/1 -> Fcn2/1
  Fcn2/1 -> Product2/1
  Divide/1 -> Product2/2
  Product2/1 -> Sum3/1
  Product/1 -> Sum3/2
  Sum3/1 -> Product3/1  "f_Thscr"
  A_floor/1 -> Product3/2
  Product3/1 -> Scope/1, Phi_airASair/1
  rho_air/1 -> [rho_air]

== system ModelGreenhouse/Cap_soil1 ==
  d : Inport
  A_floor : Inport  Port=2
  Cp_soil : Gain  Gain=1.05e3
  Product : Product
  rho_soil : Gain  Gain=1400
  Cap : Outport
  wires:
  d/1 -> Cp_soil/1
  Cp_soil/1 -> rho_soil/1
  rho_soil/1 -> Product/1
  A_floor/1 -> Product/2
  Product/1 -> Cap/1

== system ModelGreenhouse/Cap_soil2 ==
  d : Inport
  A_floor : Inport  Port=2
  Cp_soil : Gain  Gain=1.05e3
  Product : Product
  rho_soil : Gain  Gain=1400
  Cap : Outport
  wires:
  d/1 -> Cp_soil/1
  Cp_soil/1 -> rho_soil/1
  rho_soil/1 -> Product/1
  A_floor/1 -> Product/2
  Product/1 -> Cap/1

== system ModelGreenhouse/Cap_soil3 ==
  d : Inport
  A_floor : Inport  Port=2
  Cp_soil : Gain  Gain=1.05e3
  Product : Product
  rho_soil : Gain  Gain=1400
  Cap : Outport
  wires:
  d/1 -> Cp_soil/1
  Cp_soil/1 -> rho_soil/1
  rho_soil/1 -> Product/1
  A_floor/1 -> Product/2
  Product/1 -> Cap/1

== system ModelGreenhouse/Cap_soil4 ==
  d : Inport
  A_floor : Inport  Port=2
  Cp_soil : Gain  Gain=1.05e3
  Product : Product
  rho_soil : Gain  Gain=1400
  Cap : Outport
  wires:
  d/1 -> Cp_soil/1
  Cp_soil/1 -> rho_soil/1
  rho_soil/1 -> Product/1
  A_floor/1 -> Product/2
  Product/1 -> Cap/1

== system ModelGreenhouse/Cap_soil5 ==
  d : Inport
  A_floor : Inport  Port=2
  Cp_soil : Gain  Gain=1.05e3
  Product : Product
  rho_soil : Gain  Gain=1400
  Cap : Outport
  wires:
  d/1 -> Cp_soil/1
  Cp_soil/1 -> rho_soil/1
  rho_soil/1 -> Product/1
  A_floor/1 -> Product/2
  Product/1 -> Cap/1

== system ModelGreenhouse/Control - Screen ==
  I : Inport
  Constant : Constant  Value=0
  Constant1 : Constant
  Constant2 : Constant  Value=0
  Enable : Constant
  Rate Limiter : RateLimiter  RisingSlewLimit=1/1200  FallingSlewLimit=-1/1200
  Scope1 : Scope
  Switch : Switch  Criteria=u2 > Threshold  Threshold=20
  Switch1 : Switch  Criteria=u2 > Threshold
  U_Thrscr : Outport
  Reset : Outport  Port=2
  wires:
  I/1 -> Switch/2
  Constant/1 -> Switch/1
  Constant1/1 -> Switch/3
  Rate Limiter/1 -> U_Thrscr/1, Scope1/1
  Switch/1 -> Reset/1, Switch1/1
  Switch1/1 -> Rate Limiter/1
  Enable/1 -> Switch1/2
  Constant2/1 -> Switch1/3

== system ModelGreenhouse/Cover(Condensation) ==
  A_cov : Inport
  T_airAS : Inport  Port=2
  T_covin : Inport  Port=3
  C_H2O_airAS : Inport  Port=4
  rho_airAS : Inport  Port=5
  VP_SatAS : Inport  Port=6
  Bias : Bias  Bias=273.15
  Constant : Constant  Value=0
  Cp_air : Constant  Value=1.006e3
  Divide1 : Product  Inputs=*/
  Fcn : Fcn  Expr=3*abs(u)^0.33
  Fcn1 : Fcn  Expr=u^(2/3)
  LE : Constant  Value=0.89
  MATLAB Function2 : MATLAB Function  TreatAsAtomicUnit=on
  MM_H2O : Gain  Gain=18e-3
  Product1 : Product  Inputs=4
  Product2 : Product  Inputs=3
  Rate Limiter : RateLimiter  RisingSlewLimit=5  FallingSlewLimit=-200  SampleTimeMode=inherited
  Rg : Gain  Gain=8.314
  Scope2 : Scope
  Sum : Sum  Inputs=|+-
  Sum1 : Sum  Inputs=|-+
  Phi_water_cond_covin : Outport
  wires:
  T_airAS/1 -> Sum/1, Bias/1
  T_covin/1 -> Sum/2
  Sum/1 -> Fcn/1
  Bias/1 -> Rg/1
  Rg/1 -> Divide1/2
  rho_airAS/1 -> Product1/1  "rho_air"
  LE/1 -> Fcn1/1
  Fcn1/1 -> Product1/2
  Cp_air/1 -> Product1/3
  Fcn/1 -> Product1/4  "K"
  VP_SatAS/1 -> MM_H2O/1  "VP_Sat"
  MM_H2O/1 -> Divide1/1
  Divide1/1 -> MATLAB Function2/3(thres), Sum1/1  "C_H2O_Sat"
  C_H2O_airAS/1 -> Sum1/2, MATLAB Function2/4(key)  "C_H2O_air"
  Product1/1 -> Product2/1
  A_cov/1 -> Product2/2
  Sum1/1 -> Product2/3
  Constant/1 -> MATLAB Function2/2(u_lower)
  Product2/1 -> MATLAB Function2/1(u_upper)
  MATLAB Function2/1(Out) -> Rate Limiter/1
  Rate Limiter/1 -> Scope2/1, Phi_water_cond_covin/1

== system ModelGreenhouse/Cover(cov->airAS) ==
  A_cov : Inport
  Tcovin : Inport  Port=2
  TairAS : Inport  Port=3
  Fcn : Fcn  Expr=3*abs(u)^0.33
  Product : Product  Inputs=3
  Sum : Sum  Inputs=|+-
  Q_covin->air : Outport
  wires:
  Tcovin/1 -> Sum/1
  TairAS/1 -> Sum/2
  Sum/1 -> Product/2, Fcn/1
  Fcn/1 -> Product/3  "k"
  Product/1 -> Q_covin->air/1
  A_cov/1 -> Product/1

== system ModelGreenhouse/Cover(cov->sky) ==
  A_cov : Inport
  T_sky : Inport  Port=2
  T_covout : Inport  Port=3
  " Stefan-Boltzmann constant" : Constant  Value=5.67e-8
  " epsilon_cov" : Constant  Value=0.9
  Bias : Bias  Bias=273.15
  Bias1 : Bias  Bias=273.15
  Fcn : Fcn  Expr=u^4
  Fcn1 : Fcn  Expr=u^4
  Product : Product  Inputs=4
  Sum : Sum  Inputs=|+-
  R_FIR_covout->sky : Outport
  wires:
  A_cov/1 -> Product/1  "A_cov"
  T_covout/1 -> Bias/1
  T_sky/1 -> Bias1/1
  Bias/1 -> Fcn/1
  Bias1/1 -> Fcn1/1
  Fcn/1 -> Sum/1
  Fcn1/1 -> Sum/2
  Sum/1 -> Product/3
  " epsilon_cov"/1 -> Product/2
  Product/1 -> R_FIR_covout->sky/1
  " Stefan-Boltzmann constant"/1 -> Product/4

== system ModelGreenhouse/Cover(out->covout) ==
  A_cov : Inport
  Tout : Inport  Port=2
  Tcovout : Inport  Port=3
  Vwind : Inport  Port=4
  Constant : Constant  Value=4
  Fcn : Fcn  Expr=2.5 * abs(u)^0.8
  Fcn1 : Fcn  Expr=2.8 + 1.2 * abs(u)^1
  MATLAB Function1 : MATLAB Function  TreatAsAtomicUnit=on
  Product : Product  Inputs=3
  Sum : Sum  Inputs=|+-
  Q_out->covout : Outport
  wires:
  A_cov/1 -> Product/1  "A_cov"
  Tout/1 -> Sum/1
  Tcovout/1 -> Sum/2
  Sum/1 -> Product/2
  MATLAB Function1/1(Out) -> Product/3
  Product/1 -> Q_out->covout/1
  Vwind/1 -> Fcn1/1, Fcn/1, MATLAB Function1/4(key)
  Fcn/1 -> MATLAB Function1/1(u_upper)
  Fcn1/1 -> MATLAB Function1/2(u_lower)
  Constant/1 -> MATLAB Function1/3(thres)

== system ModelGreenhouse/Cover(out->in) ==
  A_cov : Inport
  lambda_cov : Inport  Port=2
  d_cov : Inport  Port=3
  T_covout : Inport  Port=4
  T_covin : Inport  Port=5
  Divide1 : Product  Inputs=*/
  Product : Product  Inputs=3
  Sum : Sum  Inputs=|+-
  Q_covout->covin : Outport
  wires:
  A_cov/1 -> Product/1  "A_cov"
  lambda_cov/1 -> Divide1/1
  d_cov/1 -> Divide1/2
  T_covout/1 -> Sum/1
  T_covin/1 -> Sum/2
  Divide1/1 -> Product/2
  Sum/1 -> Product/3
  Product/1 -> Q_covout->covin/1

== system ModelGreenhouse/FIR_can->cov ==
  note: Thre screen is from Texas
  A_Floor : Inport
  LAI : Inport  Port=2
  T_covin : Inport  Port=3
  T_can : Inport  Port=4
  U_Thrscr : Inport  Port=5
  " Stefan-Boltzmann constant" : Constant  Value=5.67e-8
  Bias : Bias  Bias=273.15
  Bias1 : Bias  Bias=273.15
  Fcn : Fcn  Expr=1 - exp(-0.94 * u)
  Fcn1 : Fcn  Expr=u^4
  Fcn2 : Fcn  Expr=u^4
  Fcn3 : Fcn  Expr=1-u
  Fcn4 : Fcn  Expr=1-u
  Product : Product
  Product1 : Product  Inputs=6
  Product2 : Product
  Sum : Sum  Inputs=|+-
  epsilon_can : Constant
  epsilon_cov : Constant  Value=0.9
  tau_cov : Constant  Value=0.11
  R_FIR_can->cov : Outport
  wires:
  LAI/1 -> Fcn/1
  A_Floor/1 -> Product/1
  Fcn/1 -> Product/2
  Fcn2/1 -> Sum/2
  Bias/1 -> Fcn1/1
  Fcn1/1 -> Sum/1
  Bias1/1 -> Fcn2/1
  Sum/1 -> Product1/6
  Product/1 -> Product1/5  "A_i"
  epsilon_cov/1 -> Product1/3
  epsilon_can/1 -> Product1/2
  " Stefan-Boltzmann constant"/1 -> Product1/1
  Product1/1 -> R_FIR_can->cov/1
  T_can/1 -> Bias/1
  T_covin/1 -> Bias1/1
  U_Thrscr/1 -> Product2/2
  tau_cov/1 -> Fcn3/1
  Fcn3/1 -> Product2/1
  Product2/1 -> Fcn4/1
  Fcn4/1 -> Product1/4

== system ModelGreenhouse/FIR_can->floor ==
  A_floor : Inport
  LAI : Inport  Port=2
  Tcan : Inport  Port=3
  Tfloor : Inport  Port=4
  " Stefan-Boltzmann constant" : Constant  Value=5.67e-8
  Bias : Bias  Bias=273.15
  Bias1 : Bias  Bias=273.15
  F : Constant
  Fcn : Fcn  Expr=1 - exp(-u)
  Fcn1 : Fcn  Expr=u^4
  Fcn2 : Fcn  Expr=u^4
  K_FIR : Gain  Gain=0.94
  Product : Product  Inputs=7
  Sum : Sum  Inputs=|+-
  epsilon_can : Constant
  epsilon_floor : Constant
  R_FIR_can->floor : Outport
  wires:
  LAI/1 -> K_FIR/1
  Fcn/1 -> Product/2
  A_floor/1 -> Product/1
  K_FIR/1 -> Fcn/1
  Product/1 -> R_FIR_can->floor/1
  epsilon_can/1 -> Product/3
  epsilon_floor/1 -> Product/4
  F/1 -> Product/5
  " Stefan-Boltzmann constant"/1 -> Product/6
  Fcn1/1 -> Sum/1
  Tfloor/1 -> Bias1/1
  Fcn2/1 -> Sum/2
  Bias1/1 -> Fcn2/1
  Tcan/1 -> Bias/1
  Bias/1 -> Fcn1/1
  Sum/1 -> Product/7

== system ModelGreenhouse/FIR_can->sky ==
  A_Floor : Inport
  LAI : Inport  Port=2
  T_sky : Inport  Port=3
  T_canopy : Inport  Port=4
  Bias : Bias  Bias=273.15
  Bias1 : Bias  Bias=273.15
  FIR transmission coefficient - cover : Constant  Value=0
  Fcn : Fcn  Expr=1 - exp(-u)
  Fcn1 : Fcn  Expr=u^4
  Fcn2 : Fcn  Expr=u^4
  K_FIR : Gain  Gain=0.94
  Product : Product  Inputs=6
  Sum : Sum  Inputs=|+-
  epsilon_can : Constant
  epsilon_sky : Constant
  R_FIR_can->sky : Outport
  wires:
  LAI/1 -> K_FIR/1
  K_FIR/1 -> Fcn/1
  A_Floor/1 -> Product/1
  Fcn/1 -> Product/2
  epsilon_can/1 -> Product/3
  epsilon_sky/1 -> Product/4
  FIR transmission coefficient - cover/1 -> Product/5  "F"
  Product/1 -> R_FIR_can->sky/1
  Fcn1/1 -> Sum/1
  Bias/1 -> Fcn1/1
  Bias1/1 -> Fcn2/1
  Fcn2/1 -> Sum/2
  T_canopy/1 -> Bias/1
  T_sky/1 -> Bias1/1
  Sum/1 -> Product/6

== system ModelGreenhouse/FIR_floor->cov ==
  note: Thre screen is from Texas
  A_Floor : Inport
  LAI : Inport  Port=2
  T_covin : Inport  Port=3
  T_floor : Inport  Port=4
  U_Thrscr : Inport  Port=5
  " Stefan-Boltzmann constant" : Constant  Value=5.67e-8
  -KFIR : Gain  Gain=-0.94
  Bias : Bias  Bias=273.15
  Bias1 : Bias  Bias=273.15
  Fcn1 : Fcn  Expr=u^4
  Fcn2 : Fcn  Expr=u^4
  Fcn3 : Fcn  Expr=1-u
  Fcn4 : Fcn  Expr=1-u
  Math Function : Math  SaturateOnIntegerOverflow=on
  Product1 : Product  Inputs=6
  Product2 : Product
  Product3 : Product
  Sum : Sum  Inputs=|+-
  epsilon_cov : Constant  Value=0.9
  epsilon_floor : Constant
  tau_cov : Constant  Value=0.11
  R_FIR_floor->cov : Outport
  wires:
  Fcn2/1 -> Sum/2
  Bias/1 -> Fcn1/1
  Fcn1/1 -> Sum/1
  Bias1/1 -> Fcn2/1
  Sum/1 -> Product1/6
  A_Floor/1 -> Product1/5  "A_i"
  epsilon_cov/1 -> Product1/3
  epsilon_floor/1 -> Product1/2
  " Stefan-Boltzmann constant"/1 -> Product1/1
  Product1/1 -> R_FIR_floor->cov/1
  LAI/1 -> -KFIR/1
  -KFIR/1 -> Math Function/1
  T_covin/1 -> Bias1/1
  T_floor/1 -> Bias/1
  tau_cov/1 -> Fcn3/1
  U_Thrscr/1 -> Product2/2
  Fcn3/1 -> Product2/1
  Product2/1 -> Fcn4/1
  Fcn4/1 -> Product3/1
  Math Function/1 -> Product3/2
  Product3/1 -> Product1/4  "F"

== system ModelGreenhouse/Floor -> Soil1 ==
  A_Floor : Inport
  T_Floor : Inport  Port=2
  T_Soil1 : Inport  Port=3
  d_floor : Inport  Port=4
  d_soil1 : Inport  Port=5
  Constant : Constant  Value=2
  Divide : Product  Inputs=*/
  Divide1 : Product  Inputs=*/
  Divide2 : Product  Inputs=*/
  Product : Product  Inputs=3
  Sum : Sum  Inputs=|++
  Sum1 : Sum  Inputs=|+-
  lambda_floor : Constant  Value=1.7
  lambda_soil : Constant  Value=0.85
  Q_floor->soil1 : Outport
  wires:
  d_floor/1 -> Divide/1
  lambda_floor/1 -> Divide/2
  d_soil1/1 -> Divide1/1
  lambda_soil/1 -> Divide1/2
  Divide/1 -> Sum/1
  Divide1/1 -> Sum/2
  Sum/1 -> Divide2/2
  Constant/1 -> Divide2/1
  T_Floor/1 -> Sum1/1
  T_Soil1/1 -> Sum1/2
  Divide2/1 -> Product/3
  A_Floor/1 -> Product/2
  Sum1/1 -> Product/1
  Product/1 -> Q_floor->soil1/1

== system ModelGreenhouse/Floor->sky ==
  note: Fix me if you wanna a FIR pass though
  A_Floor : Inport
  LAI : Inport  Port=2
  T_floor : Inport  Port=3
  T_sky : Inport  Port=4
  -K_FIR : Gain  Gain=-0.94
  Bias : Bias  Bias=273.15
  Bias1 : Bias  Bias=273.15
  Fcn : Fcn  Expr=u^4
  Fcn1 : Fcn  Expr=u^4
  Product : Product  Inputs=5
  Sum : Sum  Inputs=|+-
  epsilon_cov : Constant  Value=0.9
  epsilon_floor : Constant
  tau_FIR_cov : Gain  Gain=0
  R_FIR_floorsky : Outport
  wires:
  LAI/1 -> -K_FIR/1
  -K_FIR/1 -> tau_FIR_cov/1
  Bias1/1 -> Fcn1/1
  Bias/1 -> Fcn/1
  T_floor/1 -> Bias/1
  T_sky/1 -> Bias1/1
  Fcn/1 -> Sum/1
  Fcn1/1 -> Sum/2
  Sum/1 -> Product/5
  tau_FIR_cov/1 -> Product/4
  A_Floor/1 -> Product/1
  Product/1 -> R_FIR_floorsky/1
  epsilon_floor/1 -> Product/2
  epsilon_cov/1 -> Product/3
